simulink model "MillCircuit"  (R2017a)
settings: Solver=ode45  StartTime=0.0  StopTime=options.simulation.stoptime  RelTol=options.simulation.errortol
values from neighbouring files (symbols this model uses):
  options = struct('model_params',struct(),'initial_state',struct(),                 'control_system',struct(),'process_noise',struct(),                 'sensor_noise',struct(),'faults',struct(),                 'simulation',struct())    [params_SAGmill.m]
libraries: simulink x1
settings Model: Creator=Brandon  LastModifiedBy=Brandon
settings SolverCC: ZeroCrossAlgorithm=Adaptive
settings DataIOCC: SaveFormat=Array  SaveTime=off
settings OptimizationCC: BlockReduction=off  BooleanDataType=off  LifeSpan=inf
settings DebuggingCC: SaveWithParameterizedLinksMsg=none  UnderspecifiedInitializationDetection=Classic  MergeDetectMultiDrivingBlocksExec=none  SignalResolutionControl=TryResolveAllWithWarning  SFUnexpectedBacktrackingDiag=warning  SFNoUnconditionalDefaultTransitionDiag=warning  SFExecutionAtInitializationDiag=none
settings HardwareCC: ProdBitPerPointer=32  ProdBitPerSizeT=32  ProdBitPerPtrDiffT=32  ProdLargestAtomicFloat=None  ProdIntDivRoundTo=Undefined  ProdEndianess=Unspecified  ProdWordSize=32  ProdHWDeviceType=32-bit Generic  TargetUnknown=on
settings ModelReferenceCC: PropagateSignalLabelsOutOfModel=off
settings GRTTargetCC: TargetLangStandard=C89/C90 (ANSI)  GeneratePreprocessorConditionals=Disable all
settings ConfigComp: CovMetricSettings=dw  CovHtmlReporting=on  CovSaveCumulativeToWorkspaceVar=on  CovSaveSingleToWorkspaceVar=on  CovExternalEMLEnable=off  CovSFcnEnable=off

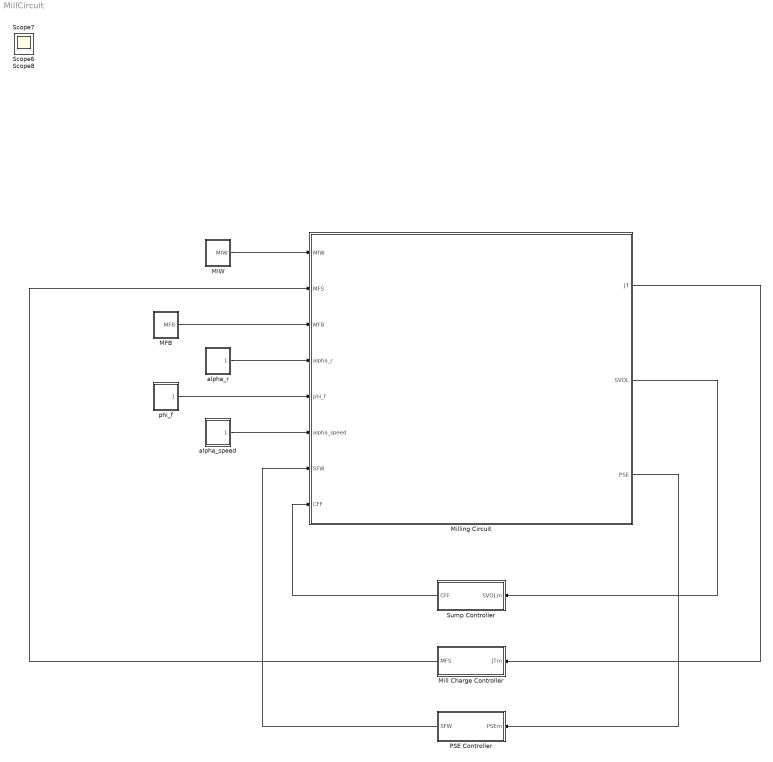
== system MillCircuit ==
  MFB : Subsystem
  MIW : Subsystem
  Mill Charge Controller : Subsystem
  Milling Circuit : Subsystem
  PSE Controller : Subsystem
  Sump Controller : Subsystem
  alpha_r : Subsystem
  alpha_speed : Subsystem
  phi_f : Subsystem
  Scope6 : Scope
  Scope7 : Scope
  Scope8 : Scope
  wires:
  MIW/1(MIW) -> Milling Circuit/1(MIW)
  MFB/1(MFB) -> Milling Circuit/3(MFB)
  alpha_speed/1(alpha_speed) -> Milling Circuit/6(alpha_speed)
  Milling Circuit/2(SVOL) -> Sump Controller/1(SVOLm)
  Milling Circuit/3(PSE) -> PSE Controller/1(PSEm)
  Milling Circuit/1(JT) -> Mill Charge Controller/1(JTm)
  Sump Controller/1(CFF) -> Milling Circuit/8(CFF)
  Mill Charge Controller/1(MFS) -> Milling Circuit/2(MFS)
  PSE Controller/1(SFW) -> Milling Circuit/7(SFW)
  alpha_r/1(alpha_r) -> Milling Circuit/4(alpha_r)
  phi_f/1(phi_f) -> Milling Circuit/5(phi_f)

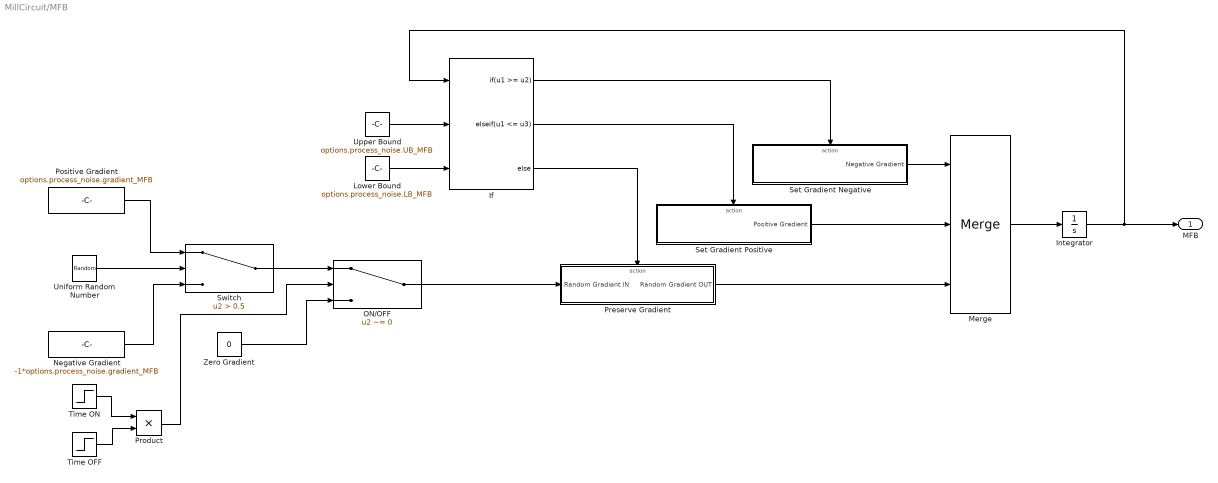
== system MillCircuit/MFB ==
  If : If  NumInputs=3  IfExpression=u1 >= u2  ElseIfExpressions=u1 <= u3  ZeroCross=off
  Integrator : Integrator  InitialCondition=options.initial_state.MFB
  Lower Bound : Constant  Value=options.process_noise.LB_MFB
  Merge : Merge  Inputs=3
  Negative Gradient : Constant  Value=-1*options.process_noise.gradient_MFB
  ON/OFF : Switch  Criteria=u2 ~= 0  Threshold=1
  Positive Gradient : Constant  Value=options.process_noise.gradient_MFB
  Preserve Gradient : Subsystem  TreatAsAtomicUnit=on
  Product : Product
  Set Gradient Negative : Subsystem  TreatAsAtomicUnit=on
  Set Gradient Positive : Subsystem  TreatAsAtomicUnit=on
  Switch : Switch  Criteria=u2 > Threshold  Threshold=0.5
  Time OFF : Step  Time=options.process_noise.time_off  Before=1  After=0  SampleTime=0
  Time ON : Step  Time=options.process_noise.time_on  SampleTime=0
  Uniform Random Number : UniformRandomNumber  Minimum=0  Seed=options.process_noise.seed_MFB  SampleTime=options.process_noise.sample_MFB
  Upper Bound : Constant  Value=options.process_noise.UB_MFB
  Zero Gradient : Constant  Value=0
  MFB : Outport
  wires:
  Uniform Random Number/1 -> Switch/2
  Positive Gradient/1 -> Switch/1
  Negative Gradient/1 -> Switch/3
  Switch/1 -> ON/OFF/1
  Zero Gradient/1 -> ON/OFF/3
  Integrator/1 -> If/1, MFB/1
  Time ON/1 -> Product/1
  Time OFF/1 -> Product/2
  Product/1 -> ON/OFF/2
  Lower Bound/1 -> If/3
  Upper Bound/1 -> If/2
  ON/OFF/1 -> Preserve Gradient/1(Random Gradient IN)
  If/3 -> Preserve Gradient/Action
  If/2 -> Set Gradient Positive/Action
  If/1 -> Set Gradient Negative/Action
  Set Gradient Negative/1(Negative Gradient) -> Merge/1
  Set Gradient Positive/1(Positive Gradient) -> Merge/2
  Preserve Gradient/1(Random Gradient OUT) -> Merge/3
  Merge/1 -> Integrator/1

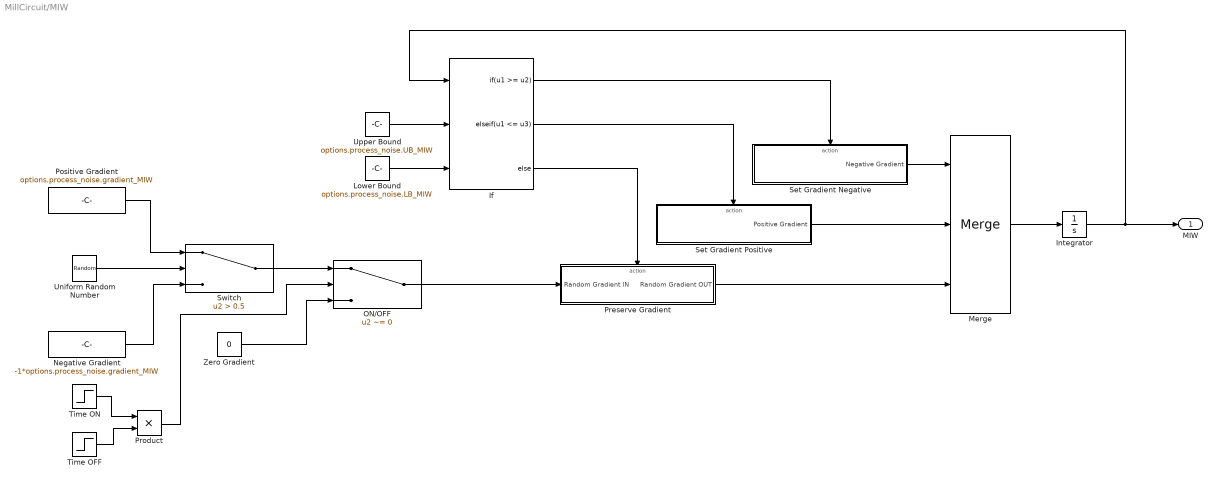
== system MillCircuit/MIW ==
  If : If  NumInputs=3  IfExpression=u1 >= u2  ElseIfExpressions=u1 <= u3  ZeroCross=off
  Integrator : Integrator  InitialCondition=options.initial_state.MIW
  Lower Bound : Constant  Value=options.process_noise.LB_MIW
  Merge : Merge  Inputs=3
  Negative Gradient : Constant  Value=-1*options.process_noise.gradient_MIW
  ON/OFF : Switch  Criteria=u2 ~= 0  Threshold=1
  Positive Gradient : Constant  Value=options.process_noise.gradient_MIW
  Preserve Gradient : Subsystem  TreatAsAtomicUnit=on
  Product : Product
  Set Gradient Negative : Subsystem  TreatAsAtomicUnit=on
  Set Gradient Positive : Subsystem  TreatAsAtomicUnit=on
  Switch : Switch  Criteria=u2 > Threshold  Threshold=0.5
  Time OFF : Step  Time=options.process_noise.time_off  Before=1  After=0  SampleTime=0
  Time ON : Step  Time=options.process_noise.time_on  SampleTime=0
  Uniform Random Number : UniformRandomNumber  Minimum=0  Seed=options.process_noise.seed_MIW  SampleTime=options.process_noise.sample_MIW
  Upper Bound : Constant  Value=options.process_noise.UB_MIW
  Zero Gradient : Constant  Value=0
  MIW : Outport
  wires:
  Uniform Random Number/1 -> Switch/2
  Positive Gradient/1 -> Switch/1
  Negative Gradient/1 -> Switch/3
  Switch/1 -> ON/OFF/1
  Zero Gradient/1 -> ON/OFF/3
  Integrator/1 -> If/1, MIW/1
  Time ON/1 -> Product/1
  Time OFF/1 -> Product/2
  Product/1 -> ON/OFF/2
  Lower Bound/1 -> If/3
  Upper Bound/1 -> If/2
  ON/OFF/1 -> Preserve Gradient/1(Random Gradient IN)
  If/3 -> Preserve Gradient/Action
  If/2 -> Set Gradient Positive/Action
  If/1 -> Set Gradient Negative/Action
  Set Gradient Negative/1(Negative Gradient) -> Merge/1
  Set Gradient Positive/1(Positive Gradient) -> Merge/2
  Preserve Gradient/1(Random Gradient OUT) -> Merge/3
  Merge/1 -> Integrator/1

== system MillCircuit/Mill Charge Controller ==
  JTm : Inport
  Controller Gain : Gain  Gain=options.control_system.K2
  Integrator : Integrator
  Intergral Time Constant : Gain  Gain=1/options.control_system.TI2
  MFSs : Constant  Value=options.initial_state.MFS
  Set Point : Constant  Value=options.control_system.JT_SP
  Signal Filter : TransferFcn  Denominator=[options.control_system.tauf2 1]
  Sum : Sum  Inputs=-+|
  Sum1 : Sum  Inputs=|++
  Sum4 : Sum  Inputs=|++
  MFS : Outport
  wires:
  MFSs/1 -> Sum4/2
  Sum4/1 -> MFS/1
  Sum/1 -> Controller Gain/1
  Integrator/1 -> Sum1/2
  Intergral Time Constant/1 -> Integrator/1
  Controller Gain/1 -> Intergral Time Constant/1, Sum1/1
  Set Point/1 -> Sum/2
  Signal Filter/1 -> Sum/1
  Sum1/1 -> Sum4/1
  JTm/1 -> Signal Filter/1

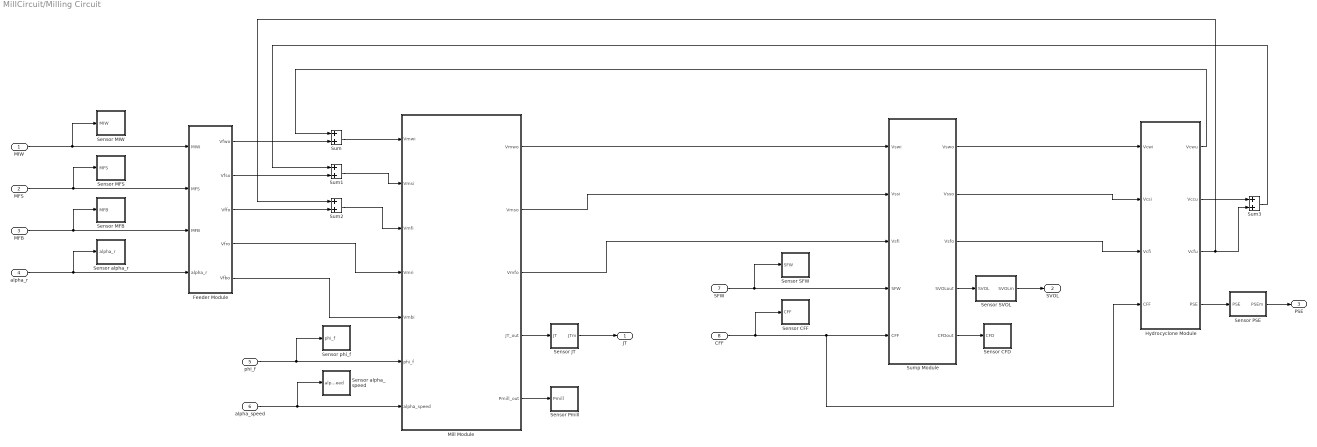
== system MillCircuit/Milling Circuit ==
  MIW : Inport
  MFS : Inport  Port=2
  MFB : Inport  Port=3
  alpha_r : Inport  Port=4
  phi_f : Inport  Port=5
  alpha_speed : Inport  Port=6
  SFW : Inport  Port=7
  CFF : Inport  Port=8
  Feeder Module : Subsystem
  Hydrocyclone Module : Subsystem
  Mill Module : Subsystem
  Sensor CFD : Subsystem
  Sensor CFF : Subsystem
  Sensor JT : Subsystem
  Sensor MFB : Subsystem
  Sensor MFS : Subsystem
  Sensor MIW : Subsystem
  Sensor PSE : Subsystem
  Sensor Pmill : Subsystem
  Sensor SFW : Subsystem
  Sensor SVOL : Subsystem
  Sensor alpha_r : Subsystem
  Sensor alpha_speed : Subsystem
  Sensor phi_f : Subsystem
  Sum{,1..3} (4 alike) : Sum
  Sump Module : Subsystem
  JT : Outport
  SVOL : Outport  Port=2
  PSE : Outport  Port=3
  wires:
  Sensor JT/1(JTm) -> JT/1
  Feeder Module/1(Vfwo) -> Sum/2
  Feeder Module/2(Vfso) -> Sum1/2
  Feeder Module/3(Vffo) -> Sum2/2
  Feeder Module/4(Vfro) -> Mill Module/4(Vmri)
  Feeder Module/5(Vfbo) -> Mill Module/5(Vmbi)
  Mill Module/1(Vmwo) -> Sump Module/1(Vswi)
  Mill Module/2(Vmso) -> Sump Module/2(Vssi)
  Mill Module/3(Vmfo) -> Sump Module/3(Vsfi)
  Sump Module/1(Vswo) -> Hydrocyclone Module/1(Vcwi)
  Sump Module/2(Vsso) -> Hydrocyclone Module/2(Vcsi)
  Sump Module/3(Vsfo) -> Hydrocyclone Module/3(Vcfi)
  Sum/1 -> Mill Module/1(Vmwi)
  Sum1/1 -> Mill Module/2(Vmsi)
  Sum2/1 -> Mill Module/3(Vmfi)
  Hydrocyclone Module/3(Vcfu) -> Sum2/1, Sum3/2
  Sum3/1 -> Sum1/1
  Hydrocyclone Module/2(Vccu) -> Sum3/1
  Hydrocyclone Module/1(Vcwu) -> Sum/1
  Sensor PSE/1(PSEm) -> PSE/1
  MIW/1 -> Sensor MIW/1(MIW), Feeder Module/1(MIW)
  MFS/1 -> Sensor MFS/1(MFS), Feeder Module/2(MFS)
  MFB/1 -> Sensor MFB/1(MFB), Feeder Module/3(MFB)
  alpha_speed/1 -> Sensor alpha_speed/1(alpha_speed), Mill Module/7(alpha_speed)
  SFW/1 -> Sump Module/4(SFW), Sensor SFW/1(SFW)
  CFF/1 -> Sensor CFF/1(CFF), Hydrocyclone Module/4(CFF), Sump Module/5(CFF)
  Sensor SVOL/1(SVOLm) -> SVOL/1
  Mill Module/4(JT_out) -> Sensor JT/1(JT)
  Mill Module/5(Pmill_out) -> Sensor Pmill/1(Pmill)
  Sump Module/4(SVOLout) -> Sensor SVOL/1(SVOL)
  Hydrocyclone Module/4(PSE) -> Sensor PSE/1(PSE)
  Sump Module/5(CFDout) -> Sensor CFD/1(CFD)
  alpha_r/1 -> Sensor alpha_r/1(alpha_r), Feeder Module/4(alpha_r)
  phi_f/1 -> Mill Module/6(phi_f), Sensor phi_f/1(phi_f)

== system MillCircuit/PSE Controller ==
  PSEm : Inport
  Controller Gain : Gain  Gain=options.control_system.K3
  Integrator : Integrator
  Intergral Time Constant : Gain  Gain=1/options.control_system.TI3
  SFWs : Constant  Value=options.initial_state.SFW
  Set Point : Constant  Value=options.control_system.PSE_SP
  Signal Filter : TransferFcn  Denominator=[options.control_system.tauf3 1]
  Sum : Sum  Inputs=-+|
  Sum1 : Sum  Inputs=|++
  Sum4 : Sum  Inputs=|++
  SFW : Outport
  wires:
  Sum1/1 -> Sum4/1
  Signal Filter/1 -> Sum/1
  Set Point/1 -> Sum/2
  Controller Gain/1 -> Sum1/1, Intergral Time Constant/1
  Intergral Time Constant/1 -> Integrator/1
  Integrator/1 -> Sum1/2
  Sum/1 -> Controller Gain/1
  Sum4/1 -> SFW/1
  SFWs/1 -> Sum4/2
  PSEm/1 -> Signal Filter/1

== system MillCircuit/Sump Controller ==
  SVOLm : Inport
  CFFs : Constant  Value=options.initial_state.CFF
  Controller Gain : Gain  Gain=-1*options.control_system.K1
  Divide : Product  Inputs=*/
  Integral Time Constant : Gain  Gain=1/options.control_system.TI1
  Integrator : Integrator
  Set Point : Constant  Value=options.control_system.SVOL_SP
  Signal Filter : TransferFcn  Denominator=[options.control_system.tauf1 1]
  Sum : Sum  Inputs=-+|
  Sum1 : Sum  Inputs=|++
  Sum4 : Sum  Inputs=|++
  Sump Crossectional Area : Constant  Value=options.model_params.Asump
  CFF : Outport
  wires:
  Signal Filter/1 -> Sum/1
  Set Point/1 -> Sum/2
  Controller Gain/1 -> Sum1/1, Integral Time Constant/1
  Integral Time Constant/1 -> Integrator/1
  Integrator/1 -> Sum1/2
  Sump Crossectional Area/1 -> Divide/2
  Sum/1 -> Divide/1
  Divide/1 -> Controller Gain/1
  Sum4/1 -> CFF/1
  CFFs/1 -> Sum4/2
  Sum1/1 -> Sum4/1
  SVOLm/1 -> Signal Filter/1

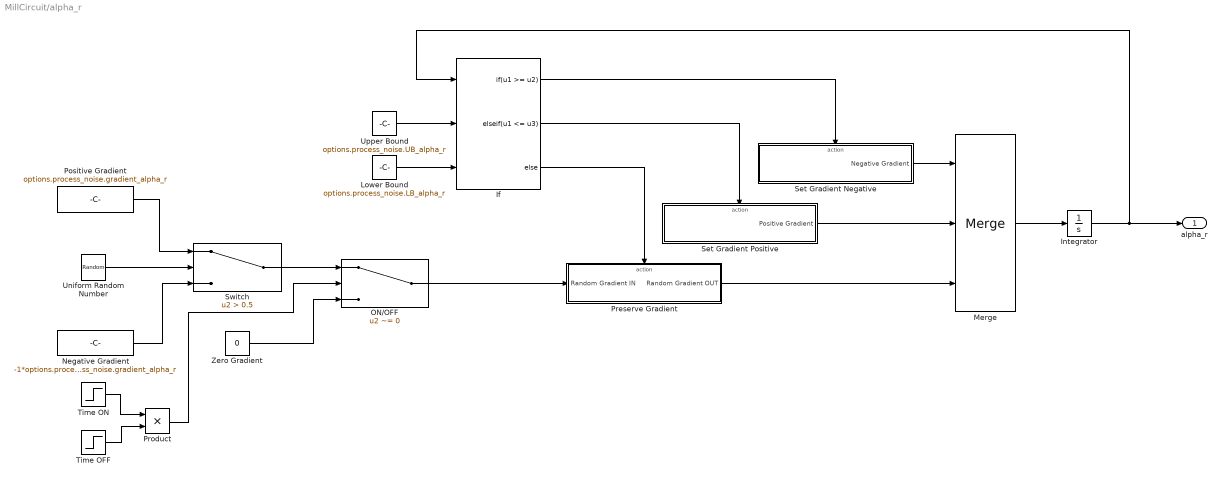
== system MillCircuit/alpha_r ==
  If : If  NumInputs=3  IfExpression=u1 >= u2  ElseIfExpressions=u1 <= u3  ZeroCross=off
  Integrator : Integrator  InitialCondition=options.model_params.alpha_r
  Lower Bound : Constant  Value=options.process_noise.LB_alpha_r
  Merge : Merge  Inputs=3
  Negative Gradient : Constant  Value=-1*options.process_noise.gradient_alpha_r
  ON/OFF : Switch  Criteria=u2 ~= 0  Threshold=1
  Positive Gradient : Constant  Value=options.process_noise.gradient_alpha_r
  Preserve Gradient : Subsystem  TreatAsAtomicUnit=on
  Product : Product
  Set Gradient Negative : Subsystem  TreatAsAtomicUnit=on
  Set Gradient Positive : Subsystem  TreatAsAtomicUnit=on
  Switch : Switch  Criteria=u2 > Threshold  Threshold=0.5
  Time OFF : Step  Time=options.process_noise.time_off  Before=1  After=0  SampleTime=0
  Time ON : Step  Time=options.process_noise.time_on  SampleTime=0
  Uniform Random Number : UniformRandomNumber  Minimum=0  Seed=options.process_noise.seed_alpha_r  SampleTime=options.process_noise.sample_alpha_r
  Upper Bound : Constant  Value=options.process_noise.UB_alpha_r
  Zero Gradient : Constant  Value=0
  alpha_r : Outport
  wires:
  Uniform Random Number/1 -> Switch/2
  Positive Gradient/1 -> Switch/1
  Negative Gradient/1 -> Switch/3
  Switch/1 -> ON/OFF/1
  Zero Gradient/1 -> ON/OFF/3
  Integrator/1 -> If/1, alpha_r/1
  Time ON/1 -> Product/1
  Time OFF/1 -> Product/2
  Product/1 -> ON/OFF/2
  Lower Bound/1 -> If/3
  Upper Bound/1 -> If/2
  ON/OFF/1 -> Preserve Gradient/1(Random Gradient IN)
  If/3 -> Preserve Gradient/Action
  If/2 -> Set Gradient Positive/Action
  If/1 -> Set Gradient Negative/Action
  Set Gradient Negative/1(Negative Gradient) -> Merge/1
  Set Gradient Positive/1(Positive Gradient) -> Merge/2
  Preserve Gradient/1(Random Gradient OUT) -> Merge/3
  Merge/1 -> Integrator/1

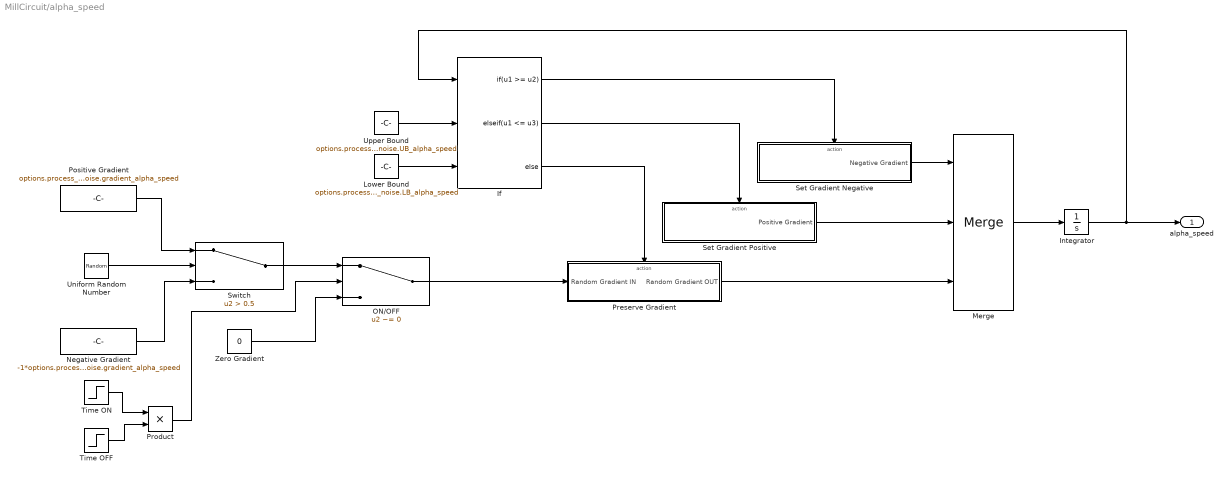
== system MillCircuit/alpha_speed ==
  If : If  NumInputs=3  IfExpression=u1 >= u2  ElseIfExpressions=u1 <= u3  ZeroCross=off
  Integrator : Integrator  InitialCondition=options.model_params.alpha_speed
  Lower Bound : Constant  Value=options.process_noise.LB_alpha_speed
  Merge : Merge  Inputs=3
  Negative Gradient : Constant  Value=-1*options.process_noise.gradient_alpha_speed
  ON/OFF : Switch  Criteria=u2 ~= 0  Threshold=1
  Positive Gradient : Constant  Value=options.process_noise.gradient_alpha_speed
  Preserve Gradient : Subsystem  TreatAsAtomicUnit=on
  Product : Product
  Set Gradient Negative : Subsystem  TreatAsAtomicUnit=on
  Set Gradient Positive : Subsystem  TreatAsAtomicUnit=on
  Switch : Switch  Criteria=u2 > Threshold  Threshold=0.5
  Time OFF : Step  Time=options.process_noise.time_off  Before=1  After=0  SampleTime=0
  Time ON : Step  Time=options.process_noise.time_on  SampleTime=0
  Uniform Random Number : UniformRandomNumber  Minimum=0  Seed=options.process_noise.seed_alpha_speed  SampleTime=options.process_noise.sample_alpha_speed
  Upper Bound : Constant  Value=options.process_noise.UB_alpha_speed
  Zero Gradient : Constant  Value=0
  alpha_speed : Outport
  wires:
  Uniform Random Number/1 -> Switch/2
  Positive Gradient/1 -> Switch/1
  Negative Gradient/1 -> Switch/3
  Switch/1 -> ON/OFF/1
  Zero Gradient/1 -> ON/OFF/3
  Integrator/1 -> If/1, alpha_speed/1
  Time ON/1 -> Product/1
  Time OFF/1 -> Product/2
  Product/1 -> ON/OFF/2
  Lower Bound/1 -> If/3
  Upper Bound/1 -> If/2
  ON/OFF/1 -> Preserve Gradient/1(Random Gradient IN)
  If/3 -> Preserve Gradient/Action
  If/2 -> Set Gradient Positive/Action
  If/1 -> Set Gradient Negative/Action
  Set Gradient Negative/1(Negative Gradient) -> Merge/1
  Set Gradient Positive/1(Positive Gradient) -> Merge/2
  Preserve Gradient/1(Random Gradient OUT) -> Merge/3
  Merge/1 -> Integrator/1

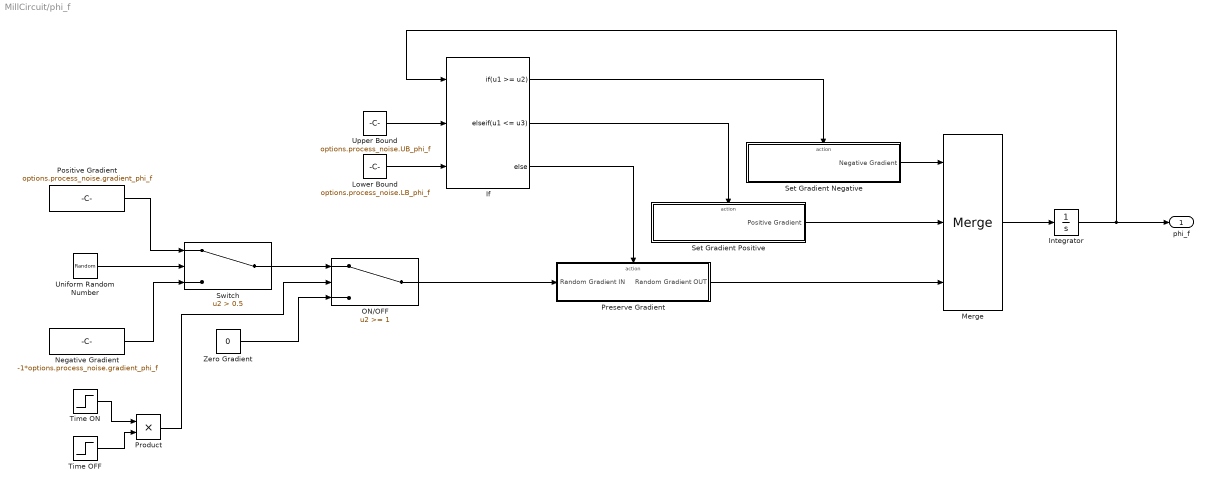
== system MillCircuit/phi_f ==
  If : If  NumInputs=3  IfExpression=u1 >= u2  ElseIfExpressions=u1 <= u3  ZeroCross=off
  Integrator : Integrator  InitialCondition=options.model_params.phi_f
  Lower Bound : Constant  Value=options.process_noise.LB_phi_f
  Merge : Merge  Inputs=3
  Negative Gradient : Constant  Value=-1*options.process_noise.gradient_phi_f
  ON/OFF : Switch  Threshold=1
  Positive Gradient : Constant  Value=options.process_noise.gradient_phi_f
  Preserve Gradient : Subsystem  TreatAsAtomicUnit=on
  Product : Product
  Set Gradient Negative : Subsystem  TreatAsAtomicUnit=on
  Set Gradient Positive : Subsystem  TreatAsAtomicUnit=on
  Switch : Switch  Criteria=u2 > Threshold  Threshold=0.5
  Time OFF : Step  Time=options.process_noise.time_off  Before=1  After=0  SampleTime=0
  Time ON : Step  Time=options.process_noise.time_on  SampleTime=0
  Uniform Random Number : UniformRandomNumber  Minimum=0  Seed=options.process_noise.seed_phi_f  SampleTime=options.process_noise.sample_phi_f
  Upper Bound : Constant  Value=options.process_noise.UB_phi_f
  Zero Gradient : Constant  Value=0
  phi_f : Outport
  wires:
  Uniform Random Number/1 -> Switch/2
  Positive Gradient/1 -> Switch/1
  Negative Gradient/1 -> Switch/3
  Switch/1 -> ON/OFF/1
  Zero Gradient/1 -> ON/OFF/3
  Integrator/1 -> If/1, phi_f/1
  Time ON/1 -> Product/1
  Time OFF/1 -> Product/2
  Product/1 -> ON/OFF/2
  Lower Bound/1 -> If/3
  Upper Bound/1 -> If/2
  ON/OFF/1 -> Preserve Gradient/1(Random Gradient IN)
  If/3 -> Preserve Gradient/Action
  If/2 -> Set Gradient Positive/Action
  If/1 -> Set Gradient Negative/Action
  Set Gradient Negative/1(Negative Gradient) -> Merge/1
  Set Gradient Positive/1(Positive Gradient) -> Merge/2
  Preserve Gradient/1(Random Gradient OUT) -> Merge/3
  Merge/1 -> Integrator/1

== system MillCircuit/MFB/Preserve Gradient ==
  Random Gradient IN : Inport
  Action Port : ActionPort  ActionType=else
  Random Gradient OUT : Outport
  wires:
  Random Gradient IN/1 -> Random Gradient OUT/1

== system MillCircuit/MFB/Set Gradient Negative ==
  Action Port : ActionPort  ActionType=then
  Negative Gradient CONST : Constant  Value=-1*options.process_noise.gradient_MFB
  Negative Gradient : Outport  InitialOutput=-1*options.process_noise.gradient_MFB
  wires:
  Negative Gradient CONST/1 -> Negative Gradient/1

== system MillCircuit/MFB/Set Gradient Positive ==
  Action Port : ActionPort  ActionType=elseif
  Positive Gradient CONST : Constant  Value=options.process_noise.gradient_MFB
  Positive Gradient : Outport  InitialOutput=options.process_noise.gradient_MFB
  wires:
  Positive Gradient CONST/1 -> Positive Gradient/1

== system MillCircuit/MIW/Preserve Gradient ==
  Random Gradient IN : Inport
  Action Port : ActionPort  ActionType=else
  Random Gradient OUT : Outport
  wires:
  Random Gradient IN/1 -> Random Gradient OUT/1

== system MillCircuit/MIW/Set Gradient Negative ==
  Action Port : ActionPort  ActionType=then
  Negative Gradient CONST : Constant  Value=-1*options.process_noise.gradient_MIW
  Negative Gradient : Outport  InitialOutput=-1*options.process_noise.gradient_MIW
  wires:
  Negative Gradient CONST/1 -> Negative Gradient/1

== system MillCircuit/MIW/Set Gradient Positive ==
  Action Port : ActionPort  ActionType=elseif
  Positive Gradient CONST : Constant  Value=options.process_noise.gradient_MIW
  Positive Gradient : Outport  InitialOutput=options.process_noise.gradient_MIW
  wires:
  Positive Gradient CONST/1 -> Positive Gradient/1

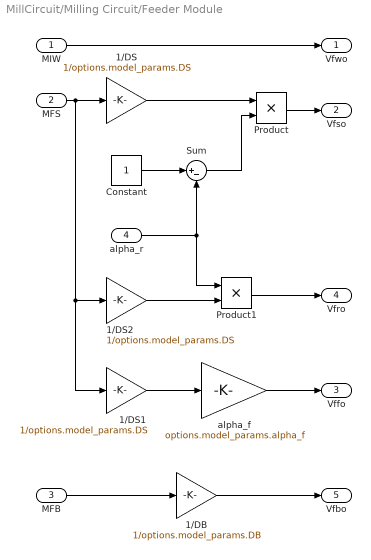
== system MillCircuit/Milling Circuit/Feeder Module ==
  MIW : Inport
  MFS : Inport  Port=2
  MFB : Inport  Port=3
  alpha_r : Inport  Port=4
  1/DB : Gain  Gain=1/options.model_params.DB
  1/DS : Gain  Gain=1/options.model_params.DS
  1/DS1 : Gain  Gain=1/options.model_params.DS
  1/DS2 : Gain  Gain=1/options.model_params.DS
  Constant : Constant
  Product : Product
  Product1 : Product
  Sum : Sum  Inputs=|+-
  alpha_f : Gain  Gain=options.model_params.alpha_f
  Vfwo : Outport
  Vfso : Outport  Port=2
  Vffo : Outport  Port=3
  Vfro : Outport  Port=4
  Vfbo : Outport  Port=5
  wires:
  MIW/1 -> Vfwo/1
  1/DS/1 -> Product/1
  1/DS1/1 -> alpha_f/1
  alpha_f/1 -> Vffo/1
  MFS/1 -> 1/DS1/1, 1/DS2/1, 1/DS/1
  1/DS2/1 -> Product1/2
  MFB/1 -> 1/DB/1
  1/DB/1 -> Vfbo/1
  alpha_r/1 -> Product1/1, Sum/2
  Constant/1 -> Sum/1
  Sum/1 -> Product/2
  Product/1 -> Vfso/1
  Product1/1 -> Vfro/1

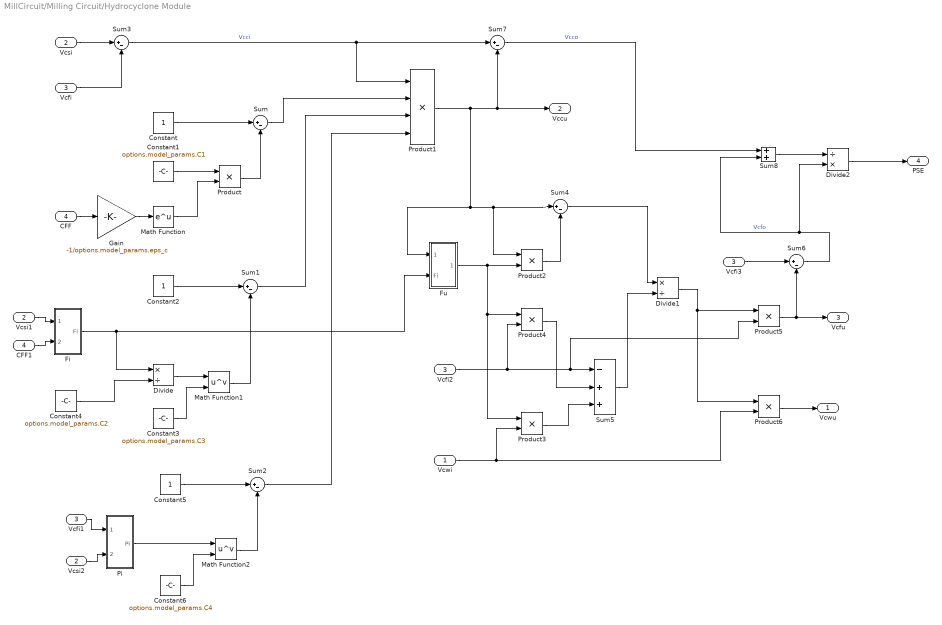
== system MillCircuit/Milling Circuit/Hydrocyclone Module ==
  Vcwi : Inport
  Vcsi : Inport  Port=2
  Vcfi : Inport  Port=3
  CFF : Inport  Port=4
  CFF1 : InportShadow  Port=4
  Constant : Constant
  Constant1 : Constant  Value=options.model_params.C1
  Constant2 : Constant
  Constant3 : Constant  Value=options.model_params.C3
  Constant4 : Constant  Value=options.model_params.C2
  Constant5 : Constant
  Constant6 : Constant  Value=options.model_params.C4
  Divide : Product  Inputs=*/
  Divide1 : Product  Inputs=*/
  Divide2 : Product  Inputs=/*
  Fi : Subsystem
  Fu : Subsystem
  Gain : Gain  Gain=-1/options.model_params.eps_c
  Math Function : Math  SaturateOnIntegerOverflow=on
  Math Function1 : Math  Operator=pow  SaturateOnIntegerOverflow=on
  Math Function2 : Math  Operator=pow  SaturateOnIntegerOverflow=on
  Pi : Subsystem
  Product{,2..6} (6 alike) : Product
  Product1 : Product  Inputs=4
  Sum{,1..4,6..7} (7 alike) : Sum  Inputs=|+-
  Sum5 : Sum  Inputs=-++
  Sum8 : Sum
  Vcfi1 : InportShadow  Port=3
  Vcfi2 : InportShadow  Port=3
  Vcfi3 : InportShadow  Port=3
  Vcsi1 : InportShadow  Port=2
  Vcsi2 : InportShadow  Port=2
  Vcwu : Outport
  Vccu : Outport  Port=2
  Vcfu : Outport  Port=3
  PSE : Outport  Port=4
  wires:
  Vcsi1/1 -> Fi/1(Vcsi)
  CFF1/1 -> Fi/2(CFF)
  Vcfi1/1 -> Pi/1(Vcfi)
  Vcsi2/1 -> Pi/2(Vcsi)
  Constant/1 -> Sum/1
  CFF/1 -> Gain/1
  Constant1/1 -> Product/1
  Math Function/1 -> Product/2
  Product/1 -> Sum/2
  Gain/1 -> Math Function/1
  Constant2/1 -> Sum1/1
  Divide/1 -> Math Function1/1
  Math Function1/1 -> Sum1/2
  Constant3/1 -> Math Function1/2
  Fi/1(Fi) -> Divide/1, Fu/2(Fi)
  Constant4/1 -> Divide/2
  Constant5/1 -> Sum2/1
  Pi/1(Pi) -> Math Function2/1
  Math Function2/1 -> Sum2/2
  Constant6/1 -> Math Function2/2
  Sum2/1 -> Product1/4
  Sum1/1 -> Product1/3
  Sum/1 -> Product1/2
  Vcsi/1 -> Sum3/1
  Vcfi/1 -> Sum3/2
  Sum3/1 -> Sum7/1, Product1/1  "Vcci"
  Product1/1 -> Sum4/1, Product2/1, Fu/1(Vccu), Vccu/1, Sum7/2
  Fu/1(Fu) -> Product3/1, Product4/1, Product2/2
  Product2/1 -> Sum4/2
  Sum4/1 -> Divide1/1
  Vcfi2/1 -> Product4/2, Product5/2, Sum5/1
  Vcwi/1 -> Product6/2, Product3/2
  Product3/1 -> Sum5/3
  Product4/1 -> Sum5/2
  Sum5/1 -> Divide1/2
  Product5/1 -> Vcfu/1, Sum6/2
  Divide1/1 -> Product6/1, Product5/1
  Product6/1 -> Vcwu/1
  Vcfi3/1 -> Sum6/1
  Sum6/1 -> Sum8/2, Divide2/2  "Vcfo"
  Sum7/1 -> Sum8/1  "Vcco"
  Sum8/1 -> Divide2/1
  Divide2/1 -> PSE/1

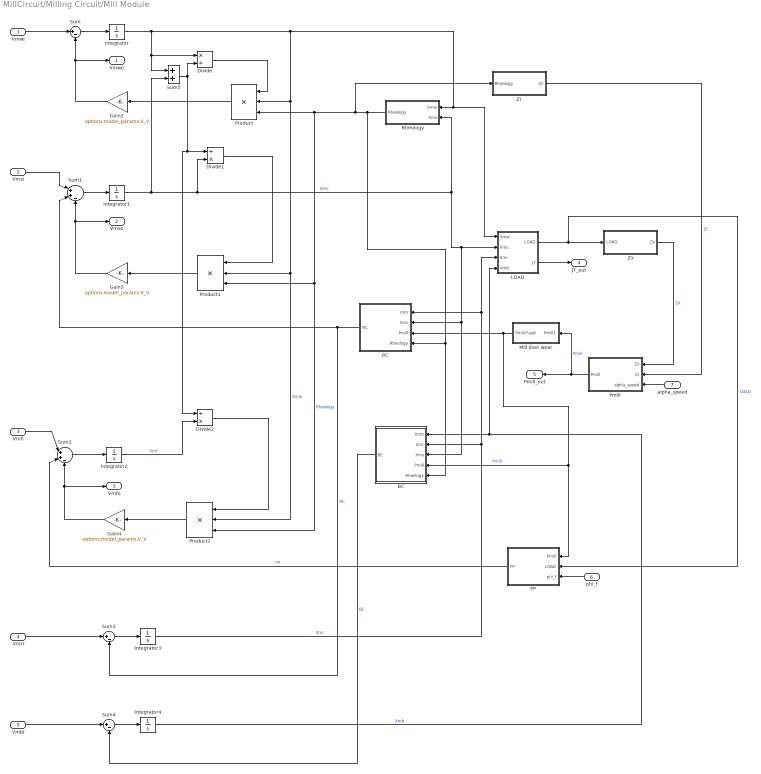
== system MillCircuit/Milling Circuit/Mill Module ==
  Vmwi : Inport
  Vmsi : Inport  Port=2
  Vmfi : Inport  Port=3
  Vmri : Inport  Port=4
  Vmbi : Inport  Port=5
  phi_f : Inport  Port=6
  alpha_speed : Inport  Port=7
  BC : Subsystem
  Divide : Product  Inputs=*/
  Divide1 : Product  Inputs=/*
  Divide2 : Product  Inputs=/*
  FP : Subsystem
  Gain2 : Gain  Gain=options.model_params.V_V
  Gain3 : Gain  Gain=options.model_params.V_V
  Gain4 : Gain  Gain=options.model_params.V_V
  Integrator : Integrator  InitialCondition=options.initial_state.Xmws  LimitOutput=on  UpperSaturationLimit=options.model_params.v_mill  LowerSaturationLimit=0
  Integrator1 : Integrator  InitialCondition=options.initial_state.Xmss  LimitOutput=on  UpperSaturationLimit=options.model_params.v_mill  LowerSaturationLimit=0
  Integrator2 : Integrator  InitialCondition=options.initial_state.Xmfs  LimitOutput=on  UpperSaturationLimit=options.model_params.v_mill  LowerSaturationLimit=0
  Integrator3 : Integrator  InitialCondition=options.initial_state.Xmrs  LimitOutput=on  UpperSaturationLimit=options.model_params.v_mill  LowerSaturationLimit=0
  Integrator4 : Integrator  InitialCondition=options.initial_state.Xmbs  LimitOutput=on  UpperSaturationLimit=options.model_params.v_mill  LowerSaturationLimit=0
  LOAD : Subsystem
  Mill liner wear : Subsystem
  Pmill : Subsystem
  Product : Product  Inputs=3
  Product1 : Product  Inputs=3
  Product2 : Product  Inputs=3
  RC : Subsystem
  Rheology : Subsystem
  Sum : Sum  Inputs=|+-
  Sum1 : Sum  Inputs=|++-
  Sum2 : Sum  Inputs=|++-
  Sum3 : Sum  Inputs=|+-
  Sum4 : Sum  Inputs=|+-
  Sum5 : Sum
  Zr : Subsystem
  Zx : Subsystem
  Vmwo : Outport
  Vmso : Outport  Port=2
  Vmfo : Outport  Port=3
  JT_out : Outport  Port=4
  Pmill_out : Outport  Port=5
  wires:
  Gain4/1 -> Sum2/3, Vmfo/1
  Gain3/1 -> Sum1/3, Vmso/1
  Gain2/1 -> Sum/2, Vmwo/1
  Vmwi/1 -> Sum/1
  Sum/1 -> Integrator/1
  Integrator/1 -> Product/2, Product1/2, Product2/2, LOAD/1(Xmw), Rheology/1(Xmw), Sum5/1, Divide/1  "Xmw"
  Vmsi/1 -> Sum1/1
  Sum1/1 -> Integrator1/1
  Integrator1/1 -> Sum5/2, LOAD/2(Xms), RC/2(Xms), BC/3(Xms), Rheology/2(Xms), Divide1/2  "Xms"
  RC/1(RC) -> Sum3/2, Sum1/2  "RC"
  Vmfi/1 -> Sum2/1
  Sum2/1 -> Integrator2/1
  Integrator2/1 -> Divide2/2  "Xmf"
  FP/1(FP) -> Sum2/2  "FP"
  Vmri/1 -> Sum3/1
  Sum3/1 -> Integrator3/1
  Integrator3/1 -> RC/1(Xmr), LOAD/3(Xmr), BC/2(Xmr)  "Xmr"
  BC/1(BC) -> Sum4/2  "BC"
  Vmbi/1 -> Sum4/1
  Sum4/1 -> Integrator4/1
  Integrator4/1 -> LOAD/4(Xmb), BC/1(Xmb)  "Xmb"
  Sum5/1 -> Divide2/1, Divide1/1, Divide/2
  Product/1 -> Gain2/1
  Divide/1 -> Product/1
  Rheology/1(Rheology) -> Zr/1(Rheology), Product1/3, Product2/3, Product/3, RC/4(Rheology), BC/5(Rheology)  "Rheology"
  Divide1/1 -> Product1/1
  Product1/1 -> Gain3/1
  Zx/1(Zx) -> Pmill/1(Zx)  "Zx"
  Zr/1(Zr) -> Pmill/2(Zr)  "Zr"
  LOAD/1(LOAD) -> Zx/1(LOAD), FP/2(LOAD)  "LOAD"
  Product2/1 -> Gain4/1
  Divide2/1 -> Product2/1
  Mill liner wear/1(Pmill Fault) -> FP/1(Pmill), BC/4(Pmill), RC/3(Pmill)  "Pmill"
  LOAD/2(JT) -> JT_out/1
  phi_f/1 -> FP/3(phi_f)
  alpha_speed/1 -> Pmill/3(alpha_speed)
  Pmill/1(Pmill) -> Mill liner wear/1(Pmill1), Pmill_out/1  "Pmill"

== system MillCircuit/Milling Circuit/Sensor CFD ==
  CFD : Inport
  CFD1 : InportShadow
  ON/OFF : Switch  Criteria=u2 ~= 0  Threshold=1
  Product1 : Product
  Random Number : RandomNumber  Variance=(options.sensor_noise.global_frac*options.initial_state.CFD)^2  Seed=options.sensor_noise.seed_CFD  SampleTime=options.simulation.sampling
  Sum1 : Sum  Inputs=|++
  Terminator : Terminator
  Time OFF : Step  Time=options.sensor_noise.time_off  Before=1  After=0  SampleTime=0
  Time ON : Step  Time=options.sensor_noise.time_on  SampleTime=0
  wires:
  Time ON/1 -> Product1/1
  Time OFF/1 -> Product1/2
  Product1/1 -> ON/OFF/2
  Random Number/1 -> Sum1/2
  CFD1/1 -> ON/OFF/3  "RAW_CFD"
  ON/OFF/1 -> Terminator/1  "CFD"
  CFD/1 -> Sum1/1  "RAW_CFD"
  Sum1/1 -> ON/OFF/1

== system MillCircuit/Milling Circuit/Sensor CFF ==
  CFF : Inport
  CFF1 : InportShadow
  ON/OFF : Switch  Criteria=u2 ~= 0  Threshold=1
  Product1 : Product
  Random Number : RandomNumber  Variance=(options.sensor_noise.global_frac*options.initial_state.CFF)^2  Seed=options.sensor_noise.seed_CFF  SampleTime=options.simulation.sampling
  Sum1 : Sum  Inputs=|++
  Terminator : Terminator
  Time OFF : Step  Time=options.sensor_noise.time_off  Before=1  After=0  SampleTime=0
  Time ON : Step  Time=options.sensor_noise.time_on  SampleTime=0
  wires:
  Time ON/1 -> Product1/1
  Time OFF/1 -> Product1/2
  Product1/1 -> ON/OFF/2
  Random Number/1 -> Sum1/2
  CFF1/1 -> ON/OFF/3  "RAW_CFF"
  ON/OFF/1 -> Terminator/1  "CFF"
  CFF/1 -> Sum1/1  "RAW_CFF"
  Sum1/1 -> ON/OFF/1

== system MillCircuit/Milling Circuit/Sensor JT ==
  JT : Inport
  Delay : TransportDelay  DelayTime=options.sensor_noise.delay_JT  InitialOutput=options.initial_state.JT  BufferSize=2048
  JT1 : InportShadow
  ON/OFF : Switch  Criteria=u2 ~= 0  Threshold=1
  Product1 : Product
  Random Number : RandomNumber  Variance=(options.sensor_noise.global_frac*options.initial_state.JT)^2  Seed=options.sensor_noise.seed_JT  SampleTime=options.simulation.sampling
  Sum1 : Sum  Inputs=|++
  Time OFF : Step  Time=options.sensor_noise.time_off  Before=1  After=0  SampleTime=0
  Time ON : Step  Time=options.sensor_noise.time_on  SampleTime=0
  JTm : Outport
  wires:
  Time ON/1 -> Product1/1
  Time OFF/1 -> Product1/2
  Product1/1 -> ON/OFF/2
  Random Number/1 -> Sum1/2
  JT1/1 -> ON/OFF/3  "RAW_JT"
  ON/OFF/1 -> JTm/1  "JT"
  JT/1 -> Sum1/1  "RAW_JT"
  Sum1/1 -> Delay/1
  Delay/1 -> ON/OFF/1

== system MillCircuit/Milling Circuit/Sensor MFB ==
  MFB : Inport
  MFB1 : InportShadow
  ON/OFF : Switch  Criteria=u2 ~= 0  Threshold=1
  Product1 : Product
  Random Number : RandomNumber  Variance=(options.sensor_noise.global_frac*options.initial_state.MFB)^2  Seed=options.sensor_noise.seed_MFB  SampleTime=options.simulation.sampling
  Sum1 : Sum  Inputs=|++
  Terminator : Terminator
  Time OFF : Step  Time=options.sensor_noise.time_off  Before=1  After=0  SampleTime=0
  Time ON : Step  Time=options.sensor_noise.time_on  SampleTime=0
  wires:
  Time ON/1 -> Product1/1
  Time OFF/1 -> Product1/2
  Product1/1 -> ON/OFF/2
  Random Number/1 -> Sum1/2
  MFB1/1 -> ON/OFF/3  "RAW_MFB"
  ON/OFF/1 -> Terminator/1  "MFB"
  MFB/1 -> Sum1/1  "RAW_MFB"
  Sum1/1 -> ON/OFF/1

== system MillCircuit/Milling Circuit/Sensor MFS ==
  MFS : Inport
  MFS1 : InportShadow
  ON/OFF : Switch  Criteria=u2 ~= 0  Threshold=1
  Product1 : Product
  Random Number : RandomNumber  Variance=(options.sensor_noise.global_frac*options.initial_state.MFS)^2  Seed=options.sensor_noise.seed_MFS  SampleTime=options.simulation.sampling
  Sum1 : Sum  Inputs=|++
  Terminator : Terminator
  Time OFF : Step  Time=options.sensor_noise.time_off  Before=1  After=0  SampleTime=0
  Time ON : Step  Time=options.sensor_noise.time_on  SampleTime=0
  wires:
  Time ON/1 -> Product1/1
  Time OFF/1 -> Product1/2
  Product1/1 -> ON/OFF/2
  Random Number/1 -> Sum1/2
  MFS1/1 -> ON/OFF/3  "RAW_MFS"
  ON/OFF/1 -> Terminator/1  "MFS"
  MFS/1 -> Sum1/1  "RAW_MFS"
  Sum1/1 -> ON/OFF/1

== system MillCircuit/Milling Circuit/Sensor MIW ==
  MIW : Inport
  MIW1 : InportShadow
  ON/OFF : Switch  Criteria=u2 ~= 0  Threshold=1
  Product1 : Product
  Random Number : RandomNumber  Variance=(options.sensor_noise.global_frac*options.initial_state.MIW)^2  Seed=options.sensor_noise.seed_MIW  SampleTime=options.simulation.sampling
  Sum1 : Sum  Inputs=|++
  Terminator : Terminator
  Time OFF : Step  Time=options.sensor_noise.time_off  Before=1  After=0  SampleTime=0
  Time ON : Step  Time=options.sensor_noise.time_on  SampleTime=0
  wires:
  Time ON/1 -> Product1/1
  Time OFF/1 -> Product1/2
  Product1/1 -> ON/OFF/2
  Random Number/1 -> Sum1/2
  MIW1/1 -> ON/OFF/3  "RAW_MIW"
  ON/OFF/1 -> Terminator/1  "MIW"
  MIW/1 -> Sum1/1  "RAW_MIW"
  Sum1/1 -> ON/OFF/1

== system MillCircuit/Milling Circuit/Sensor PSE ==
  PSE : Inport
  Delay : TransportDelay  DelayTime=options.sensor_noise.delay_PSE  InitialOutput=options.initial_state.PSE  BufferSize=2048
  ON/OFF : Switch  Criteria=u2 ~= 0  Threshold=1
  PSE1 : InportShadow
  Product1 : Product
  Random Number : RandomNumber  Variance=(options.sensor_noise.global_frac*options.initial_state.PSE)^2  Seed=options.sensor_noise.seed_PSE  SampleTime=options.simulation.sampling
  Sensor Fault : Subsystem
  Sum1 : Sum  Inputs=|++
  Time OFF : Step  Time=options.sensor_noise.time_off  Before=1  After=0  SampleTime=0
  Time ON : Step  Time=options.sensor_noise.time_on  SampleTime=0
  PSEm : Outport
  wires:
  Time ON/1 -> Product1/1
  Time OFF/1 -> Product1/2
  Product1/1 -> ON/OFF/2
  Random Number/1 -> Sum1/2
  PSE1/1 -> ON/OFF/3  "RAW_PSE"
  Sensor Fault/1(PSE Faulty) -> PSEm/1  "PSE"
  PSE/1 -> Sum1/1, Sensor Fault/1(RAW_PSE)  "RAW_PSE"
  Sum1/1 -> Delay/1
  Delay/1 -> ON/OFF/1
  ON/OFF/1 -> Sensor Fault/2(PSE1)

== system MillCircuit/Milling Circuit/Sensor Pmill ==
  Pmill : Inport
  ON/OFF : Switch  Criteria=u2 ~= 0  Threshold=1
  Pmill1 : InportShadow
  Product1 : Product
  Random Number : RandomNumber  Variance=(options.sensor_noise.global_frac*options.initial_state.Pmill)^2  Seed=options.sensor_noise.seed_Pmill  SampleTime=options.simulation.sampling
  Sum1 : Sum  Inputs=|++
  Terminator : Terminator
  Time OFF : Step  Time=options.sensor_noise.time_off  Before=1  After=0  SampleTime=0
  Time ON : Step  Time=options.sensor_noise.time_on  SampleTime=0
  wires:
  Time ON/1 -> Product1/1
  Time OFF/1 -> Product1/2
  Product1/1 -> ON/OFF/2
  Random Number/1 -> Sum1/2
  Pmill1/1 -> ON/OFF/3  "RAW_Pmill"
  ON/OFF/1 -> Terminator/1  "Pmill"
  Pmill/1 -> Sum1/1  "RAW_Pmill"
  Sum1/1 -> ON/OFF/1

== system MillCircuit/Milling Circuit/Sensor SFW ==
  SFW : Inport
  ON/OFF : Switch  Criteria=u2 ~= 0  Threshold=1
  Product1 : Product
  Random Number : RandomNumber  Variance=(options.sensor_noise.global_frac*options.initial_state.SFW)^2  Seed=options.sensor_noise.seed_SFW  SampleTime=options.simulation.sampling
  SFW1 : InportShadow
  Sum1 : Sum  Inputs=|++
  Terminator : Terminator
  Time OFF : Step  Time=options.sensor_noise.time_off  Before=1  After=0  SampleTime=0
  Time ON : Step  Time=options.sensor_noise.time_on  SampleTime=0
  wires:
  Time ON/1 -> Product1/1
  Time OFF/1 -> Product1/2
  Product1/1 -> ON/OFF/2
  Random Number/1 -> Sum1/2
  SFW1/1 -> ON/OFF/3  "RAW_SFW"
  ON/OFF/1 -> Terminator/1  "SFW"
  SFW/1 -> Sum1/1  "RAW_SFW"
  Sum1/1 -> ON/OFF/1

== system MillCircuit/Milling Circuit/Sensor SVOL ==
  SVOL : Inport
  ON/OFF : Switch  Criteria=u2 ~= 0  Threshold=1
  Product1 : Product
  Random Number : RandomNumber  Variance=(options.sensor_noise.global_frac*options.model_params.SVOL)^2  Seed=options.sensor_noise.seed_SVOL  SampleTime=options.simulation.sampling
  SVOL1 : InportShadow
  Sum1 : Sum  Inputs=|++
  Time OFF : Step  Time=options.sensor_noise.time_off  Before=1  After=0  SampleTime=0
  Time ON : Step  Time=options.sensor_noise.time_on  SampleTime=0
  SVOLm : Outport
  wires:
  Time ON/1 -> Product1/1
  Time OFF/1 -> Product1/2
  Product1/1 -> ON/OFF/2
  Random Number/1 -> Sum1/2
  SVOL1/1 -> ON/OFF/3  "RAW_SVOL"
  ON/OFF/1 -> SVOLm/1  "SVOL"
  SVOL/1 -> Sum1/1  "RAW_SVOL"
  Sum1/1 -> ON/OFF/1

== system MillCircuit/Milling Circuit/Sensor alpha_r ==
  alpha_r : Inport
  ON/OFF : Switch  Criteria=u2 ~= 0  Threshold=1
  Product1 : Product
  Random Number : RandomNumber  Variance=(options.sensor_noise.global_frac*options.model_params.alpha_r)^2  Seed=options.sensor_noise.seed_alpha_r  SampleTime=options.simulation.sampling
  Sum1 : Sum  Inputs=|++
  Terminator : Terminator
  Time OFF : Step  Time=options.sensor_noise.time_off  Before=1  After=0  SampleTime=0
  Time ON : Step  Time=options.sensor_noise.time_on  SampleTime=0
  alpha_r1 : InportShadow
  wires:
  Time ON/1 -> Product1/1
  Time OFF/1 -> Product1/2
  Product1/1 -> ON/OFF/2
  Random Number/1 -> Sum1/2
  alpha_r1/1 -> ON/OFF/3  "RAW_alpha_r"
  ON/OFF/1 -> Terminator/1  "alpha_r"
  alpha_r/1 -> Sum1/1  "RAW_alpha_r"
  Sum1/1 -> ON/OFF/1

== system MillCircuit/Milling Circuit/Sensor alpha_speed ==
  alpha_speed : Inport
  ON/OFF : Switch  Criteria=u2 ~= 0  Threshold=1
  Product1 : Product
  Random Number : RandomNumber  Variance=(options.sensor_noise.global_frac*options.model_params.alpha_speed)^2  Seed=options.sensor_noise.seed_alpha_speed  SampleTime=options.simulation.sampling
  Sum1 : Sum  Inputs=|++
  Terminator : Terminator
  Time OFF : Step  Time=options.sensor_noise.time_off  Before=1  After=0  SampleTime=0
  Time ON : Step  Time=options.sensor_noise.time_on  SampleTime=0
  alpha_speed1 : InportShadow
  wires:
  Time ON/1 -> Product1/1
  Time OFF/1 -> Product1/2
  Product1/1 -> ON/OFF/2
  Random Number/1 -> Sum1/2
  alpha_speed1/1 -> ON/OFF/3  "RAW_alpha_speed"
  ON/OFF/1 -> Terminator/1  "alpha_speed"
  alpha_speed/1 -> Sum1/1  "RAW_alpha_speed"
  Sum1/1 -> ON/OFF/1

== system MillCircuit/Milling Circuit/Sensor phi_f ==
  phi_f : Inport
  Delay : TransportDelay  DelayTime=options.sensor_noise.delay_phi_f  InitialOutput=options.model_params.phi_f  BufferSize=2048
  ON/OFF : Switch  Criteria=u2 ~= 0  Threshold=1
  Product1 : Product
  Random Number : RandomNumber  Variance=(options.sensor_noise.global_frac*options.model_params.phi_f)^2  Seed=options.sensor_noise.seed_phi_f  SampleTime=options.simulation.sampling
  Sum1 : Sum  Inputs=|++
  Terminator : Terminator
  Time OFF : Step  Time=options.sensor_noise.time_off  Before=1  After=0  SampleTime=0
  Time ON : Step  Time=options.sensor_noise.time_on  SampleTime=0
  phi_f1 : InportShadow
  wires:
  Time ON/1 -> Product1/1
  Time OFF/1 -> Product1/2
  Product1/1 -> ON/OFF/2
  Random Number/1 -> Sum1/2
  phi_f1/1 -> ON/OFF/3  "RAW_phi_f"
  ON/OFF/1 -> Terminator/1  "phi_f"
  phi_f/1 -> Sum1/1  "RAW_phi_f"
  Sum1/1 -> Delay/1
  Delay/1 -> ON/OFF/1

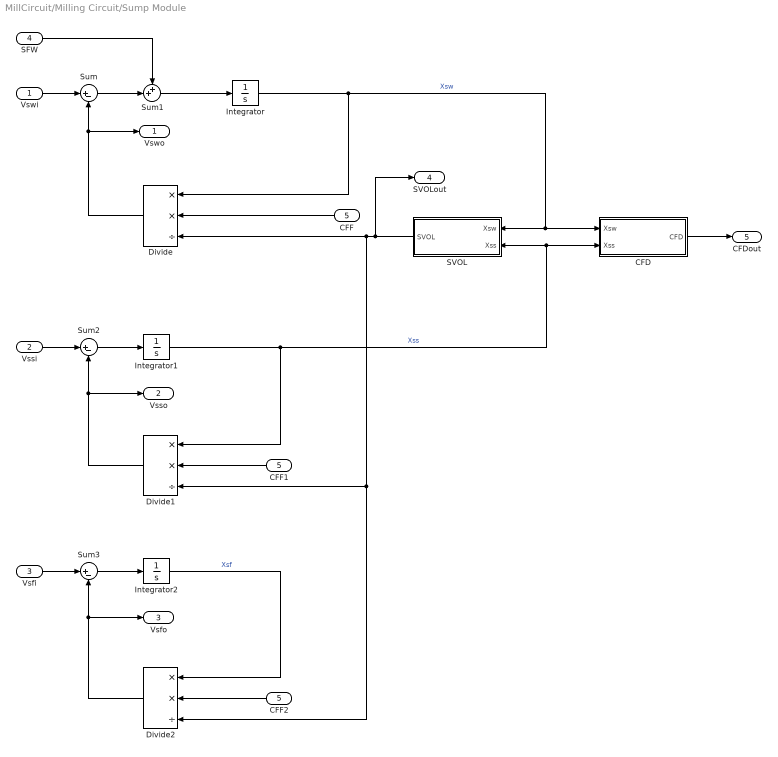
== system MillCircuit/Milling Circuit/Sump Module ==
  Vswi : Inport
  Vssi : Inport  Port=2
  Vsfi : Inport  Port=3
  SFW : Inport  Port=4
  CFF : Inport  Port=5
  CFD : Subsystem
  CFF1 : InportShadow  Port=5
  CFF2 : InportShadow  Port=5
  Divide : Product  Inputs=**/
  Divide1 : Product  Inputs=**/
  Divide2 : Product  Inputs=**/
  Integrator : Integrator  InitialCondition=options.initial_state.Xsws  LimitOutput=on  UpperSaturationLimit=2*options.model_params.SVOL  LowerSaturationLimit=0
  Integrator1 : Integrator  InitialCondition=options.initial_state.Xsss  LimitOutput=on  UpperSaturationLimit=2*options.model_params.SVOL  LowerSaturationLimit=0
  Integrator2 : Integrator  InitialCondition=options.initial_state.Xsfs  LimitOutput=on  UpperSaturationLimit=2*options.model_params.SVOL  LowerSaturationLimit=0
  SVOL : Subsystem
  Sum : Sum  Inputs=|+-
  Sum1 : Sum  Inputs=++|
  Sum2 : Sum  Inputs=|+-
  Sum3 : Sum  Inputs=|+-
  Vswo : Outport
  Vsso : Outport  Port=2
  Vsfo : Outport  Port=3
  SVOLout : Outport  Port=4
  CFDout : Outport  Port=5
  wires:
  Vswi/1 -> Sum/1
  Divide/1 -> Sum/2, Vswo/1
  Sum/1 -> Sum1/2
  SFW/1 -> Sum1/1
  Sum1/1 -> Integrator/1
  Integrator/1 -> CFD/1(Xsw), SVOL/1(Xsw), Divide/1  "Xsw"
  Vssi/1 -> Sum2/1
  Divide1/1 -> Sum2/2, Vsso/1
  Sum2/1 -> Integrator1/1
  Divide2/1 -> Vsfo/1, Sum3/2
  Sum3/1 -> Integrator2/1
  Integrator2/1 -> Divide2/1  "Xsf"
  Vsfi/1 -> Sum3/1
  CFF/1 -> Divide/2
  SVOL/1(SVOL) -> Divide1/3, Divide2/3, Divide/3, SVOLout/1
  CFF1/1 -> Divide1/2
  CFF2/1 -> Divide2/2
  Integrator1/1 -> CFD/2(Xss), SVOL/2(Xss), Divide1/1  "Xss"
  CFD/1(CFD) -> CFDout/1

== system MillCircuit/alpha_r/Preserve Gradient ==
  Random Gradient IN : Inport
  Action Port : ActionPort  ActionType=else
  Random Gradient OUT : Outport
  wires:
  Random Gradient IN/1 -> Random Gradient OUT/1

== system MillCircuit/alpha_r/Set Gradient Negative ==
  Action Port : ActionPort  ActionType=then
  Negative Gradient CONST : Constant  Value=-1*options.process_noise.gradient_alpha_r
  Negative Gradient : Outport  InitialOutput=-1*options.process_noise.gradient_alpha_r
  wires:
  Negative Gradient CONST/1 -> Negative Gradient/1

== system MillCircuit/alpha_r/Set Gradient Positive ==
  Action Port : ActionPort  ActionType=elseif
  Positive Gradient CONST : Constant  Value=options.process_noise.gradient_alpha_r
  Positive Gradient : Outport  InitialOutput=options.process_noise.gradient_alpha_r
  wires:
  Positive Gradient CONST/1 -> Positive Gradient/1

== system MillCircuit/alpha_speed/Preserve Gradient ==
  Random Gradient IN : Inport
  Action Port : ActionPort  ActionType=else
  Random Gradient OUT : Outport
  wires:
  Random Gradient IN/1 -> Random Gradient OUT/1

== system MillCircuit/alpha_speed/Set Gradient Negative ==
  Action Port : ActionPort  ActionType=then
  Negative Gradient CONST : Constant  Value=-1*options.process_noise.gradient_alpha_speed
  Negative Gradient : Outport  InitialOutput=-1*options.process_noise.gradient_alpha_speed
  wires:
  Negative Gradient CONST/1 -> Negative Gradient/1

== system MillCircuit/alpha_speed/Set Gradient Positive ==
  Action Port : ActionPort  ActionType=elseif
  Positive Gradient CONST : Constant  Value=options.process_noise.gradient_alpha_speed
  Positive Gradient : Outport  InitialOutput=options.process_noise.gradient_alpha_speed
  wires:
  Positive Gradient CONST/1 -> Positive Gradient/1

== system MillCircuit/phi_f/Preserve Gradient ==
  Random Gradient IN : Inport
  Action Port : ActionPort  ActionType=else
  Random Gradient OUT : Outport
  wires:
  Random Gradient IN/1 -> Random Gradient OUT/1

== system MillCircuit/phi_f/Set Gradient Negative ==
  Action Port : ActionPort  ActionType=then
  Negative Gradient CONST : Constant  Value=-1*options.process_noise.gradient_phi_f
  Negative Gradient : Outport  InitialOutput=-1*options.process_noise.gradient_phi_f
  wires:
  Negative Gradient CONST/1 -> Negative Gradient/1

== system MillCircuit/phi_f/Set Gradient Positive ==
  Action Port : ActionPort  ActionType=elseif
  Positive Gradient CONST : Constant  Value=options.process_noise.gradient_phi_f
  Positive Gradient : Outport  InitialOutput=options.process_noise.gradient_phi_f
  wires:
  Positive Gradient CONST/1 -> Positive Gradient/1

== system MillCircuit/Milling Circuit/Hydrocyclone Module/Fi ==
  Vcsi : Inport
  CFF : Inport  Port=2
  Divide : Product  Inputs=*/
  Fi : Outport
  wires:
  Vcsi/1 -> Divide/1
  CFF/1 -> Divide/2
  Divide/1 -> Fi/1

== system MillCircuit/Milling Circuit/Hydrocyclone Module/Fu ==
  Vccu : Inport
  Fi : Inport  Port=2
  Constant : Constant  Value=0.6
  Constant1 : Constant  Value=0.6
  Gain : Gain  Gain=1/options.model_params.eps_c
  Gain1 : Gain  Gain=1/options.model_params.alpha_su
  Gain2 : Gain  Gain=-1
  Math Function : Math  SaturateOnIntegerOverflow=on
  Product : Product
  Sum : Sum  Inputs=+-
  Sum1 : Sum  Inputs=|+-
  Fu : Outport
  wires:
  Vccu/1 -> Gain2/1
  Constant/1 -> Sum/1
  Product/1 -> Sum/2
  Constant1/1 -> Sum1/1
  Fi/1 -> Sum1/2
  Sum1/1 -> Product/1
  Gain/1 -> Gain1/1
  Gain2/1 -> Gain/1
  Gain1/1 -> Math Function/1
  Math Function/1 -> Product/2
  Sum/1 -> Fu/1

== system MillCircuit/Milling Circuit/Hydrocyclone Module/Pi ==
  Vcfi : Inport
  Vcsi : Inport  Port=2
  Divide : Product  Inputs=*/
  Pi : Outport
  wires:
  Divide/1 -> Pi/1
  Vcsi/1 -> Divide/2
  Vcfi/1 -> Divide/1

== system MillCircuit/Milling Circuit/Mill Module/BC ==
  Xmb : Inport
  Xmr : Inport  Port=2
  Xms : Inport  Port=3
  Pmill : Inport  Port=4
  Rheology : Inport  Port=5
  Divide : Product  Inputs=*/
  Gain1 : Gain  Gain=1/options.model_params.phi_b
  Gain2 : Gain  Gain=options.model_params.DS
  Gain3 : Gain  Gain=options.model_params.DB
  Product : Product
  Product1 : Product
  Sum : Sum
  Sum1 : Sum
  BC : Outport
  wires:
  Product1/1 -> BC/1
  Gain1/1 -> Product1/2
  Divide/1 -> Product1/1
  Product/1 -> Gain1/1
  Rheology/1 -> Product/2
  Pmill/1 -> Product/1
  Sum1/1 -> Divide/2
  Xms/1 -> Sum/2
  Xmr/1 -> Sum/1
  Xmb/1 -> Divide/1, Gain3/1
  Sum/1 -> Gain2/1
  Gain3/1 -> Sum1/1
  Gain2/1 -> Sum1/2

== system MillCircuit/Milling Circuit/Mill Module/FP ==
  Pmill : Inport
  LOAD : Inport  Port=2
  phi_f : Inport  Port=3
  Constant : Constant  Value=options.model_params.v_Pmax
  Constant1 : Constant
  Divide : Product  Inputs=*/
  Gain : Gain  Gain=1/options.model_params.v_mill
  Gain1 : Gain  Gain=options.model_params.alpha_phif
  Gain2 : Gain  Gain=options.model_params.DS
  Product : Product
  Sum : Sum  Inputs=|+-
  Sum1 : Sum  Inputs=++|
  FP : Outport
  wires:
  LOAD/1 -> Gain/1
  Gain/1 -> Sum/1
  Constant/1 -> Sum/2
  Sum/1 -> Gain1/1
  Constant1/1 -> Sum1/1
  Gain1/1 -> Sum1/2
  Sum1/1 -> Gain2/1
  Gain2/1 -> Product/1
  Product/1 -> Divide/2
  Pmill/1 -> Divide/1
  Divide/1 -> FP/1
  phi_f/1 -> Product/2

== system MillCircuit/Milling Circuit/Mill Module/LOAD ==
  Xmw : Inport
  Xms : Inport  Port=2
  Xmr : Inport  Port=3
  Xmb : Inport  Port=4
  Constant : Constant  Value=options.model_params.v_mill
  Divide : Product  Inputs=*/
  Saturation : Saturate  UpperLimit=options.model_params.v_mill  LowerLimit=0
  Sum : Sum  Inputs=++++
  LOAD : Outport
  JT : Outport  Port=2
  wires:
  Xmb/1 -> Sum/4
  Xms/1 -> Sum/3
  Xmr/1 -> Sum/2
  Xmw/1 -> Sum/1
  Saturation/1 -> Divide/1, LOAD/1
  Constant/1 -> Divide/2
  Divide/1 -> JT/1
  Sum/1 -> Saturation/1

== system MillCircuit/Milling Circuit/Mill Module/Mill liner wear ==
  Pmill1 : Inport
  Constant : Constant  Value=options.initial_state.Pmill
  Fault Active : Gain  Gain=options.faults.liner
  Gradient : simulink/Sources/Ramp  slope=options.faults.liner_powerloss_gradient  start=options.faults.liner_time_on  X0=0
  Max Power Loss : Gain  Gain=options.faults.liner_powerloss
  ON/OFF : Switch  Criteria=u2 ~= 0  Threshold=1
  Pmill : InportShadow
  Product : Product
  Product1 : Product
  Saturation : Saturate  UpperLimit=1  LowerLimit=0
  Sum1 : Sum  Inputs=-+|
  Time OFF : Step  Time=options.faults.liner_time_off  Before=1  After=0  SampleTime=0
  Time ON : Step  Time=options.faults.liner_time_on  SampleTime=0
  Pmill Fault : Outport
  wires:
  Pmill/1 -> Sum1/2
  Max Power Loss/1 -> Product/1
  Product/1 -> Sum1/1
  Gradient/1 -> Saturation/1
  Time ON/1 -> Product1/1
  Time OFF/1 -> Product1/2
  Product1/1 -> Fault Active/1
  Fault Active/1 -> ON/OFF/2
  Sum1/1 -> ON/OFF/1
  Pmill1/1 -> ON/OFF/3
  ON/OFF/1 -> Pmill Fault/1
  Saturation/1 -> Product/2
  Constant/1 -> Max Power Loss/1

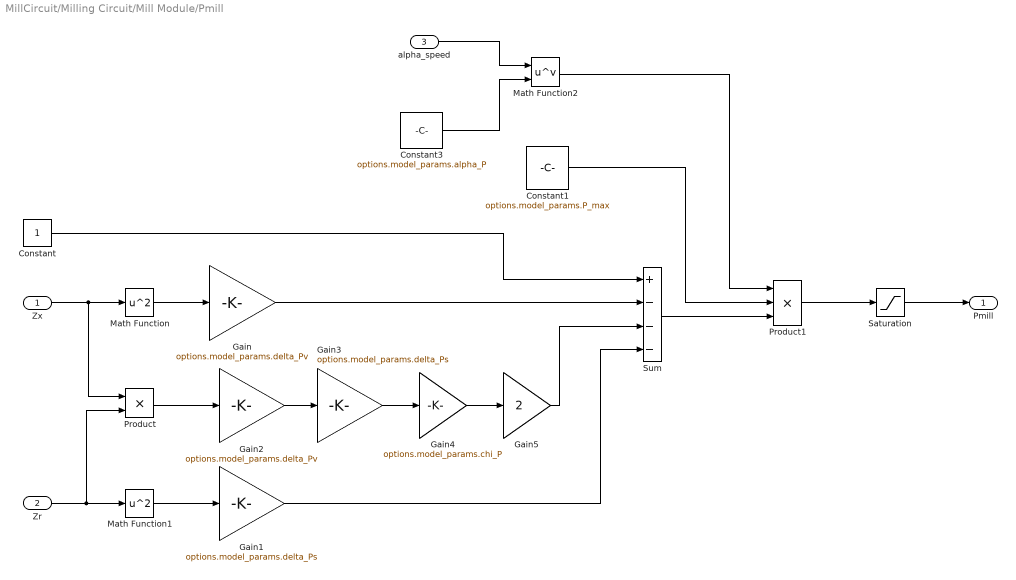
== system MillCircuit/Milling Circuit/Mill Module/Pmill ==
  Zx : Inport
  Zr : Inport  Port=2
  alpha_speed : Inport  Port=3
  Constant : Constant
  Constant1 : Constant  Value=options.model_params.P_max
  Constant3 : Constant  Value=options.model_params.alpha_P
  Gain : Gain  Gain=options.model_params.delta_Pv
  Gain1 : Gain  Gain=options.model_params.delta_Ps
  Gain2 : Gain  Gain=options.model_params.delta_Pv
  Gain3 : Gain  Gain=options.model_params.delta_Ps
  Gain4 : Gain  Gain=options.model_params.chi_P
  Gain5 : Gain  Gain=2
  Math Function : Math  Operator=square  SaturateOnIntegerOverflow=on
  Math Function1 : Math  Operator=square  SaturateOnIntegerOverflow=on
  Math Function2 : Math  Operator=pow  SaturateOnIntegerOverflow=on
  Product : Product
  Product1 : Product  Inputs=3
  Saturation : Saturate  UpperLimit=options.model_params.P_max  LowerLimit=0
  Sum : Sum  Inputs=+---
  Pmill : Outport
  wires:
  Zx/1 -> Product/1, Math Function/1
  Zr/1 -> Math Function1/1, Product/2
  Product/1 -> Gain2/1
  Math Function1/1 -> Gain1/1
  Math Function/1 -> Gain/1
  Gain2/1 -> Gain3/1
  Gain3/1 -> Gain4/1
  Gain4/1 -> Gain5/1
  Constant/1 -> Sum/1
  Gain/1 -> Sum/2
  Gain5/1 -> Sum/3
  Gain1/1 -> Sum/4
  Sum/1 -> Product1/3
  Constant1/1 -> Product1/2
  alpha_speed/1 -> Math Function2/1
  Constant3/1 -> Math Function2/2
  Math Function2/1 -> Product1/1
  Product1/1 -> Saturation/1
  Saturation/1 -> Pmill/1

== system MillCircuit/Milling Circuit/Mill Module/RC ==
  Xmr : Inport
  Xms : Inport  Port=2
  Pmill : Inport  Port=3
  Rheology : Inport  Port=4
  Divide : Product  Inputs=*/
  Gain : Gain  Gain=1/options.model_params.DS
  Gain1 : Gain  Gain=1/options.model_params.phi_r
  Product : Product
  Product1 : Product
  Sum : Sum
  RC : Outport
  wires:
  Xmr/1 -> Divide/1, Sum/1
  Xms/1 -> Sum/2
  Sum/1 -> Divide/2
  Pmill/1 -> Product/1
  Rheology/1 -> Product/2
  Product/1 -> Gain/1
  Gain/1 -> Gain1/1
  Divide/1 -> Product1/1
  Gain1/1 -> Product1/2
  Product1/1 -> RC/1

== system MillCircuit/Milling Circuit/Mill Module/Rheology ==
  Xmw : Inport
  Xms : Inport  Port=2
  Constant : Constant  Value=0.5
  Constant1 : Constant  Value=0
  Constant2 : Constant
  Divide : Product  Inputs=*/
  Math Function : Math  Operator=pow  SaturateOnIntegerOverflow=on
  Math Function1 : Math  Operator=reciprocal  SaturateOnIntegerOverflow=on
  Product : Product
  Saturation : Saturate  UpperLimit=1  LowerLimit=0
  Sum : Sum  Inputs=|+-
  Sum1 : Sum  Inputs=|+-
  eps_sv : Constant  Value=options.model_params.eps_sv
  max : MinMax  Function=max  Inputs=2
  Rheology : Outport
  wires:
  max/1 -> Math Function/1
  Math Function/1 -> Saturation/1
  Constant/1 -> Math Function/2
  Constant1/1 -> max/1
  Sum/1 -> max/2
  Constant2/1 -> Sum/1, Sum1/2
  Xms/1 -> Divide/1
  Xmw/1 -> Divide/2
  Divide/1 -> Product/2
  eps_sv/1 -> Math Function1/1
  Math Function1/1 -> Sum1/1
  Sum1/1 -> Product/1
  Product/1 -> Sum/2
  Saturation/1 -> Rheology/1

== system MillCircuit/Milling Circuit/Mill Module/Zr ==
  Rheology : Inport
  Constant : Constant
  Gain : Gain  Gain=1/options.model_params.rhe_Pmax
  Sum : Sum  Inputs=|+-
  Zr : Outport
  wires:
  Sum/1 -> Zr/1
  Constant/1 -> Sum/2
  Gain/1 -> Sum/1
  Rheology/1 -> Gain/1

== system MillCircuit/Milling Circuit/Mill Module/Zx ==
  LOAD : Inport
  Constant : Constant
  Gain : Gain  Gain=1/options.model_params.v_mill
  Gain1 : Gain  Gain=1/options.model_params.v_Pmax
  Sum : Sum  Inputs=|+-
  Zx : Outport
  wires:
  LOAD/1 -> Gain/1
  Gain/1 -> Gain1/1
  Gain1/1 -> Sum/1
  Constant/1 -> Sum/2
  Sum/1 -> Zx/1

== system MillCircuit/Milling Circuit/Sensor PSE/Sensor Fault ==
  RAW_PSE : Inport
  PSE1 : Inport  Port=2
  Bias : Gain  Gain=options.faults.PSE_sensor_bias
  Fault Active : Gain  Gain=options.faults.PSE_sensor
  ON/OFF : Switch  Criteria=u2 ~= 0  Threshold=1
  PSE : InportShadow  Port=2
  Product1 : Product
  Sum1 : Sum  Inputs=++|
  Time OFF : Step  Time=options.faults.PSE_time_off  Before=1  After=0  SampleTime=0
  Time ON : Step  Time=options.faults.PSE_time_on  SampleTime=0
  PSE Faulty : Outport
  wires:
  PSE1/1 -> ON/OFF/3
  PSE/1 -> Sum1/2
  Sum1/1 -> ON/OFF/1
  Bias/1 -> Sum1/1
  ON/OFF/1 -> PSE Faulty/1
  Time ON/1 -> Product1/1
  Time OFF/1 -> Product1/2
  Product1/1 -> Fault Active/1
  Fault Active/1 -> ON/OFF/2
  RAW_PSE/1 -> Bias/1

== system MillCircuit/Milling Circuit/Sump Module/CFD ==
  Xsw : Inport
  Xss : Inport  Port=2
  Divide : Product  Inputs=*/
  Gain : Gain  Gain=options.model_params.DS
  Sum : Sum
  Sum1 : Sum
  Xss1 : InportShadow  Port=2
  Xsw1 : InportShadow
  CFD : Outport
  wires:
  Sum/1 -> Divide/2
  Xss/1 -> Sum/2
  Xsw/1 -> Sum/1
  Xss1/1 -> Gain/1
  Gain/1 -> Sum1/2
  Xsw1/1 -> Sum1/1
  Sum1/1 -> Divide/1
  Divide/1 -> CFD/1

== system MillCircuit/Milling Circuit/Sump Module/SVOL ==
  Xsw : Inport
  Xss : Inport  Port=2
  Saturation : Saturate  UpperLimit=2*options.model_params.SVOL  LowerLimit=0
  Sum : Sum
  SVOL : Outport
  wires:
  Xsw/1 -> Sum/1
  Xss/1 -> Sum/2
  Sum/1 -> Saturation/1
  Saturation/1 -> SVOL/1
